simulink model "fixed_sch_Sample_HardThreshold"  (R2020a)
settings: Solver=VariableStepAuto  StartTime=0  StopTime=180  RelTol=1e-3
model workspace (MAT data in the model file):
  a = 0
values from neighbouring files (symbols this model uses):
  fs = 30000    [fixed_sch_run_Sample_HardThreshold.m]
  refractory = 10^-3    (= 0.001)    [fixed_sch_run_Sample_HardThreshold.m]
  th = [-20]    [fixed_sch_run_Sample_HardThreshold.m]
libraries: dsparch4 x2, simulink x2, dspswit3 x1, hdlsllib x1
settings Model: SimulationMode=accelerator  Creator=sbuccelli  LastModifiedBy=diflo

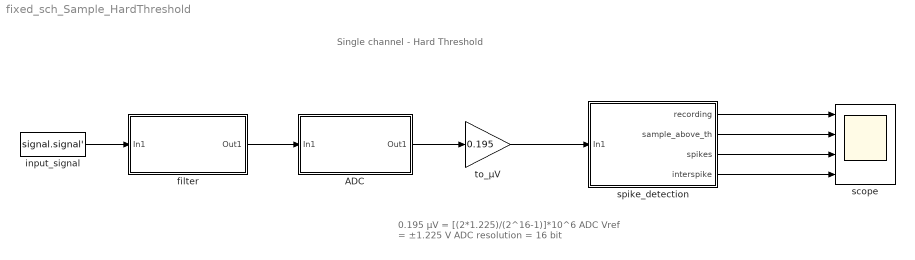
== system fixed_sch_Sample_HardThreshold ==
  note: Single channel - Hard Threshold
  note: 0.195 µV = [(2*1.225)/(2^16-1)]*10^6
      | ADC Vref = ±1.225 V
      | ADC resolution = 16 bit
  ADC : Subsystem
  filter : Subsystem
  input_signal : FromWorkspace  VariableName=signal.signal'  SampleTime=1/fs
  scope : Scope  NumInputPorts=4
  spike_detection : Subsystem
  to_µV : Gain  Gain=0.195  SaturateOnIntegerOverflow=on  OutDataTypeStr=Inherit: Same as input  ParamDataTypeStr=Inherit: Same as input
  wires:
  spike_detection/1(recording) -> scope/1
  spike_detection/2(sample_above_th) -> scope/2
  spike_detection/3(spikes) -> scope/3
  spike_detection/4(interspike) -> scope/4
  input_signal/1 -> filter/1(In1)
  filter/1(Out1) -> ADC/1(In1)
  ADC/1(Out1) -> to_µV/1
  to_µV/1 -> spike_detection/1(In1)

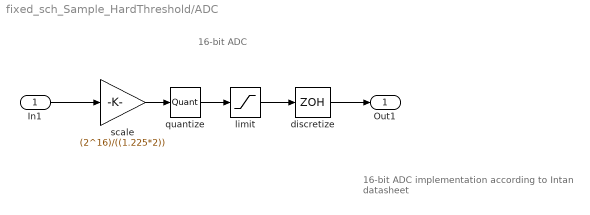
== system fixed_sch_Sample_HardThreshold/ADC ==
  note: 16-bit ADC
  note: 16-bit ADC implementation according to
      | Intan datasheet
  In1 : Inport
  discretize : ZeroOrderHold  SampleTime=-1
  limit : Saturate  UpperLimit=32767  LowerLimit=-32768
  quantize : Quantizer  QuantizationInterval=0.000000195
  scale : Gain  Gain=(2^16)/((1.225*2))  SaturateOnIntegerOverflow=on  OutDataTypeStr=Inherit: Same as input  ParamDataTypeStr=Inherit: Same as input
  Out1 : Outport
  wires:
  quantize/1 -> limit/1
  limit/1 -> discretize/1
  scale/1 -> quantize/1
  In1/1 -> scale/1
  discretize/1 -> Out1/1

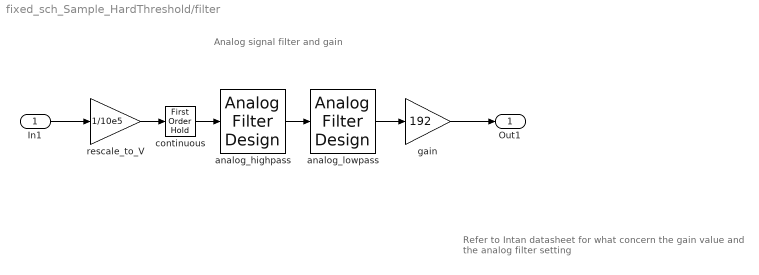
== system fixed_sch_Sample_HardThreshold/filter ==
  note: Analog signal filter and gain
  note: Refer to Intan datasheet for what concern the
      | gain value and the analog filter setting
  In1 : Inport
  analog_highpass : dsparch4/Analog Filter Design  method=Butterworth  filttype=Highpass  N=1  Wlo=300  Whi=80  Rp=2  Rs=40
  analog_lowpass : dsparch4/Analog Filter Design  method=Butterworth  filttype=Lowpass  N=3  Wlo=3000  Whi=80  Rp=2  Rs=40
  continuous : FirstOrderHold  ErrorTolerance=inf
  gain : Gain  Gain=192  SaturateOnIntegerOverflow=on  OutDataTypeStr=Inherit: Same as input  ParamDataTypeStr=Inherit: Same as input
  rescale_to_V : Gain  Gain=1/10e5
  Out1 : Outport
  wires:
  analog_lowpass/1 -> gain/1
  rescale_to_V/1 -> continuous/1
  continuous/1 -> analog_highpass/1
  gain/1 -> Out1/1
  analog_highpass/1 -> analog_lowpass/1
  In1/1 -> rescale_to_V/1

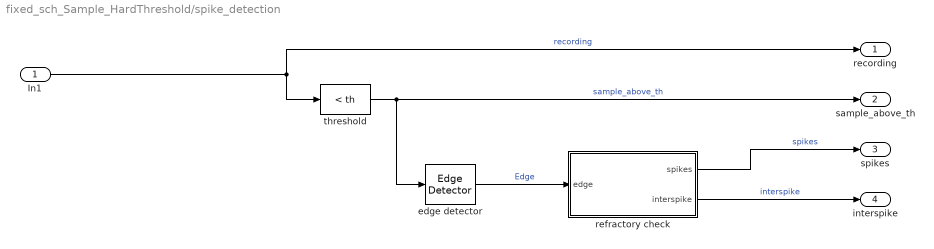
== system fixed_sch_Sample_HardThreshold/spike_detection ==
  In1 : Inport
  "edge detector " : dspswit3/Edge Detector  InputProcessing=Columns as channels (frame based)
      settings: SourceProductBaseCode=DS
  refractory check : Subsystem
  threshold : simulink/Logic and Bit Operations/Compare To Constant  relop=<  const=th  OutDataTypeStr=boolean
  recording : Outport
  sample_above_th : Outport  Port=2
  spikes : Outport  Port=3
  interspike : Outport  Port=4
  wires:
  In1/1 -> recording/1, threshold/1  "recording"
  refractory check/1(spikes) -> spikes/1  "spikes"
  threshold/1 -> sample_above_th/1, "edge detector "/1  "sample_above_th"
  refractory check/2(interspike) -> interspike/1  "interspike"
  "edge detector "/1 -> refractory check/1("edge  ")  "Edge"

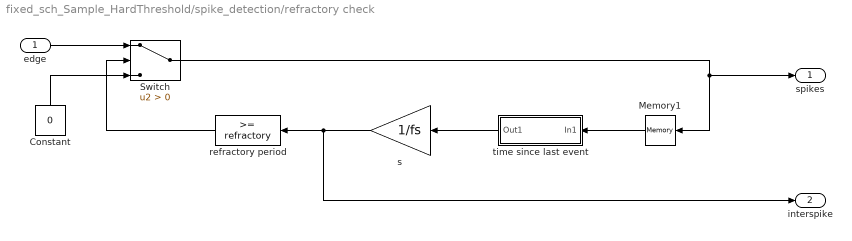
== system fixed_sch_Sample_HardThreshold/spike_detection/refractory check ==
  "edge  " : Inport
  Constant : Constant  Value=0
  Memory1 : Memory  InheritSampleTime=on
  Switch : Switch  Criteria=u2 > Threshold
  refractory period : simulink/Logic and Bit Operations/Compare To Constant  relop=>=  const=refractory  OutDataTypeStr=boolean
  s : Gain  Gain=1/fs  ParamDataTypeStr=double
  time since last event : Subsystem
  spikes : Outport
  interspike : Outport  Port=2
  wires:
  "edge  "/1 -> Switch/1
  Memory1/1 -> time since last event/1(In1)
  time since last event/1(Out1) -> s/1
  Constant/1 -> Switch/3
  s/1 -> refractory period/1, interspike/1
  Switch/1 -> spikes/1, Memory1/1
  refractory period/1 -> Switch/2

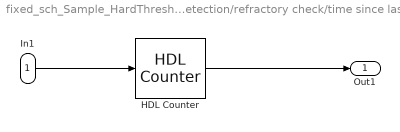
== system fixed_sch_Sample_HardThreshold/spike_detection/refractory check/time since last event ==
  In1 : Inport
  HDL Counter : hdlsllib/Sources/HDL Counter  CountType=Free running  CountInit=1  CountStep=1  CountMax=25  CountFromType=Initial value  CountFrom=1  CountResetPort=on  CountLoadPort=off  CountEnbPort=off  CountDirPort=off  CountDataType=Unsigned  CountWordLen=32  CountFracLen=0  CountSampTime=1
  Out1 : Outport
  wires:
  In1/1 -> HDL Counter/1
  HDL Counter/1 -> Out1/1
